simulink library "tenneco_lib"  (R2016b)
settings: Solver=ode45  StartTime=0.0  StopTime=10.0  RelTol=1e-3
undefined symbols (not defined in the file): Com_cntAMBInitTO_c, Com_cntAMBStopTO_c, Com_cntEC1InitTO_c, Com_cntEC1StopTO_c, Com_swAMBRx_c, Com_swEC1Rx_c, Com_swUseSPN108_c, Com_swUseSPN543_c, const, Env_pAmbPDflt_c, Env_pAmbPKOff_c, Env_pAmbPOvrd_c, Env_swAmbPOvrd_c, MSG_INIT_TIMEOUT, MSG_NOT_RECEIVED, MSG_RECEIVED_NOW, MSG_STOP_TIMEOUT
libraries: simulink x19, tenneco_lib x2
(part 2 of 5)

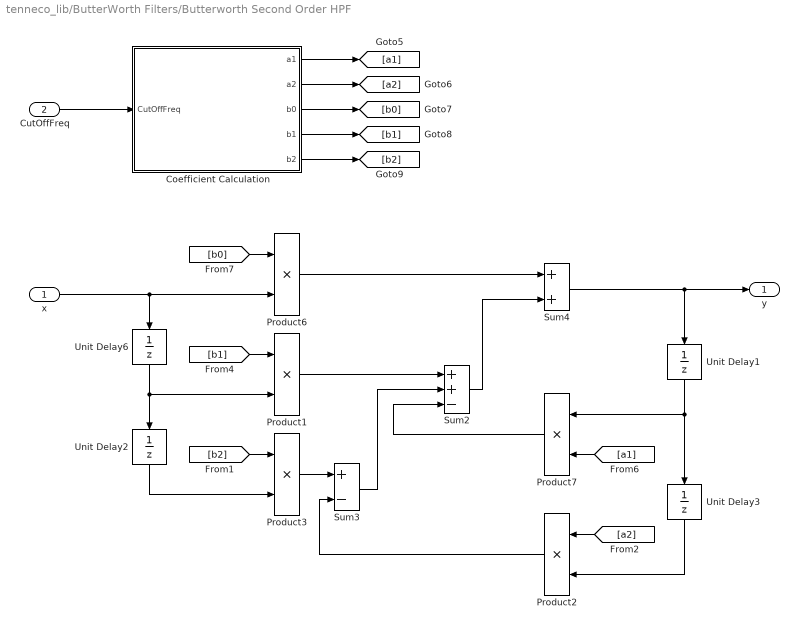
== system tenneco_lib/ButterWorth Filters/Butterworth Second Order HPF ==
  x : Inport  mask(Standard Inport){Port=1}
      mask prompts: Port "Simulink:blkprm_prompts:InOutportPortNum"
      mask help: Provide an input port for subsystems.
      mask TypeOptions Port: Port
  CutOffFreq : Inport  Port=2  mask(Standard Inport){Port=2}
      mask prompts: Port "Simulink:blkprm_prompts:InOutportPortNum"
      mask help: Provide an input port for subsystems.
      mask TypeOptions Port: Port
  Coefficient Calculation : Subsystem
  Product1 : Product  Inputs=**  InputSameDT=on  mask(Product){Inputs=**}
      mask prompts: Inputs "List of signs:"
      mask help:
      | Multiply or divide inputs.  Specify one of the following:
      |  a) * or / for each input port. For example, **/* performs the operation 'u1*u2/u3*u4'.
      |  b) scalar specifies the number of input ports to be multiplied.
      mask TypeOptions Inputs: Inputs
  Product2 : Product  Inputs=**  InputSameDT=on  mask(Product){Inputs=**}
      mask prompts: Inputs "List of signs:"
      mask help:
      | Multiply or divide inputs.  Specify one of the following:
      |  a) * or / for each input port. For example, **/* performs the operation 'u1*u2/u3*u4'.
      |  b) scalar specifies the number of input ports to be multiplied.
      mask TypeOptions Inputs: Inputs
  Product3 : Product  Inputs=**  InputSameDT=on  mask(Product){Inputs=**}
      mask prompts: Inputs "List of signs:"
      mask help:
      | Multiply or divide inputs.  Specify one of the following:
      |  a) * or / for each input port. For example, **/* performs the operation 'u1*u2/u3*u4'.
      |  b) scalar specifies the number of input ports to be multiplied.
      mask TypeOptions Inputs: Inputs
  Product6 : Product  Inputs=**  InputSameDT=on  mask(Product){Inputs=**}
      mask prompts: Inputs "List of signs:"
      mask help:
      | Multiply or divide inputs.  Specify one of the following:
      |  a) * or / for each input port. For example, **/* performs the operation 'u1*u2/u3*u4'.
      |  b) scalar specifies the number of input ports to be multiplied.
      mask TypeOptions Inputs: Inputs
  Product7 : Product  Inputs=**  InputSameDT=on  mask(Product){Inputs=**}
      mask prompts: Inputs "List of signs:"
      mask help:
      | Multiply or divide inputs.  Specify one of the following:
      |  a) * or / for each input port. For example, **/* performs the operation 'u1*u2/u3*u4'.
      |  b) scalar specifies the number of input ports to be multiplied.
      mask TypeOptions Inputs: Inputs
  Sum2 : Sum  Inputs=++-  InputSameDT=on  mask(Sum){Inputs=++-}
      mask prompts: Inputs "Simulink:blkprm_prompts:SumListofSigns"
      mask help:
      | Add or subtract inputs.  Specify one of the following:
      | a) character vector containing + or - for each input port, | for spacer between ports (e.g. ++|-|++)
      | b) scalar, >= 1, specifies the number of input ports to be summed.
      | When there is only one input port, add or subtract elements over all dimensions or one specified dimension
      mask TypeOptions Inputs: Inputs
  Sum3 : Sum  Inputs=+-  InputSameDT=on  mask(Sum){Inputs=+-}
      mask prompts: Inputs "Simulink:blkprm_prompts:SumListofSigns"
      mask help:
      | Add or subtract inputs.  Specify one of the following:
      | a) character vector containing + or - for each input port, | for spacer between ports (e.g. ++|-|++)
      | b) scalar, >= 1, specifies the number of input ports to be summed.
      | When there is only one input port, add or subtract elements over all dimensions or one specified dimension
      mask TypeOptions Inputs: Inputs
  Sum4 : Sum  InputSameDT=on  mask(Sum){Inputs=++}
      mask prompts: Inputs "Simulink:blkprm_prompts:SumListofSigns"
      mask help:
      | Add or subtract inputs.  Specify one of the following:
      | a) character vector containing + or - for each input port, | for spacer between ports (e.g. ++|-|++)
      | b) scalar, >= 1, specifies the number of input ports to be summed.
      | When there is only one input port, add or subtract elements over all dimensions or one specified dimension
      mask TypeOptions Inputs: Inputs
  Unit Delay1 : UnitDelay  InitialCondition=InitialCondition  SampleTime=-1  mask(Unit Delay){InitialCondition=0}
      mask prompts: InitialCondition "Simulink:blkprm_prompts:DelayBlkInitCond"
      mask help: Sample and hold with one sample period delay.
      mask TypeOptions InitialCondition: InitialCondition
  Unit Delay2 : UnitDelay  InitialCondition=InitialCondition  SampleTime=-1  mask(Unit Delay){InitialCondition=0}
      mask prompts: InitialCondition "Simulink:blkprm_prompts:DelayBlkInitCond"
      mask help: Sample and hold with one sample period delay.
      mask TypeOptions InitialCondition: InitialCondition
  Unit Delay3 : UnitDelay  InitialCondition=InitialCondition  SampleTime=-1  mask(Unit Delay){InitialCondition=0}
      mask prompts: InitialCondition "Simulink:blkprm_prompts:DelayBlkInitCond"
      mask help: Sample and hold with one sample period delay.
      mask TypeOptions InitialCondition: InitialCondition
  Unit Delay6 : UnitDelay  InitialCondition=InitialCondition  SampleTime=-1  mask(Unit Delay){InitialCondition=0}
      mask prompts: InitialCondition "Simulink:blkprm_prompts:DelayBlkInitCond"
      mask help: Sample and hold with one sample period delay.
      mask TypeOptions InitialCondition: InitialCondition
  y : Outport  mask(Standard Outport){Port=1}
      mask prompts: Port "Simulink:blkprm_prompts:InOutportPortNum"
      mask help: Provide an output port for subsystems.
      mask TypeOptions Port: Port
  wires:
  Unit Delay3/1 -> Product2/2
  Product2/1 -> Sum3/2
  [a2] -> Product2/1
  Sum3/1 -> Sum2/2
  Product3/1 -> Sum3/1
  Product7/1 -> Sum2/3
  Unit Delay2/1 -> Product3/2
  [b2] -> Product3/1
  Coefficient Calculation/5(b2) -> [b2]
  Coefficient Calculation/2(a2) -> [a2]
  CutOffFreq/1 -> Coefficient Calculation/1(CutOffFreq)
  x/1 -> Product6/2, Unit Delay6/1
  Coefficient Calculation/1(a1) -> [a1]
  Coefficient Calculation/4(b1) -> [b1]
  Coefficient Calculation/3(b0) -> [b0]
  Product6/1 -> Sum4/1
  Unit Delay6/1 -> Unit Delay2/1, Product1/2
  [b1] -> Product1/1
  [b0] -> Product6/1
  Product1/1 -> Sum2/1
  Sum2/1 -> Sum4/2
  [a1] -> Product7/2
  Unit Delay1/1 -> Product7/1, Unit Delay3/1
  Sum4/1 -> y/1, Unit Delay1/1

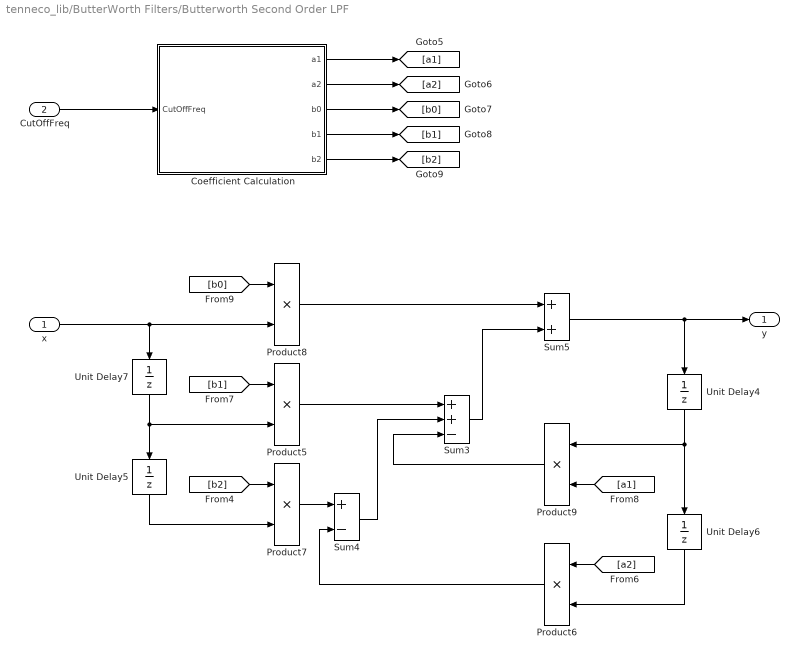
== system tenneco_lib/ButterWorth Filters/Butterworth Second Order LPF ==
  x : Inport  mask(Standard Inport){Port=1}
      mask prompts: Port "Simulink:blkprm_prompts:InOutportPortNum"
      mask help: Provide an input port for subsystems.
      mask TypeOptions Port: Port
  CutOffFreq : Inport  Port=2  mask(Standard Inport){Port=2}
      mask prompts: Port "Simulink:blkprm_prompts:InOutportPortNum"
      mask help: Provide an input port for subsystems.
      mask TypeOptions Port: Port
  Coefficient Calculation : Subsystem
  Product5 : Product  Inputs=**  InputSameDT=on  mask(Product){Inputs=**}
      mask prompts: Inputs "List of signs:"
      mask help:
      | Multiply or divide inputs.  Specify one of the following:
      |  a) * or / for each input port. For example, **/* performs the operation 'u1*u2/u3*u4'.
      |  b) scalar specifies the number of input ports to be multiplied.
      mask TypeOptions Inputs: Inputs
  Product6 : Product  Inputs=**  InputSameDT=on  mask(Product){Inputs=**}
      mask prompts: Inputs "List of signs:"
      mask help:
      | Multiply or divide inputs.  Specify one of the following:
      |  a) * or / for each input port. For example, **/* performs the operation 'u1*u2/u3*u4'.
      |  b) scalar specifies the number of input ports to be multiplied.
      mask TypeOptions Inputs: Inputs
  Product7 : Product  Inputs=**  InputSameDT=on  mask(Product){Inputs=**}
      mask prompts: Inputs "List of signs:"
      mask help:
      | Multiply or divide inputs.  Specify one of the following:
      |  a) * or / for each input port. For example, **/* performs the operation 'u1*u2/u3*u4'.
      |  b) scalar specifies the number of input ports to be multiplied.
      mask TypeOptions Inputs: Inputs
  Product8 : Product  Inputs=**  InputSameDT=on  mask(Product){Inputs=**}
      mask prompts: Inputs "List of signs:"
      mask help:
      | Multiply or divide inputs.  Specify one of the following:
      |  a) * or / for each input port. For example, **/* performs the operation 'u1*u2/u3*u4'.
      |  b) scalar specifies the number of input ports to be multiplied.
      mask TypeOptions Inputs: Inputs
  Product9 : Product  Inputs=**  InputSameDT=on  mask(Product){Inputs=**}
      mask prompts: Inputs "List of signs:"
      mask help:
      | Multiply or divide inputs.  Specify one of the following:
      |  a) * or / for each input port. For example, **/* performs the operation 'u1*u2/u3*u4'.
      |  b) scalar specifies the number of input ports to be multiplied.
      mask TypeOptions Inputs: Inputs
  Sum3 : Sum  Inputs=++-  InputSameDT=on  mask(Sum){Inputs=++-}
      mask prompts: Inputs "Simulink:blkprm_prompts:SumListofSigns"
      mask help:
      | Add or subtract inputs.  Specify one of the following:
      | a) character vector containing + or - for each input port, | for spacer between ports (e.g. ++|-|++)
      | b) scalar, >= 1, specifies the number of input ports to be summed.
      | When there is only one input port, add or subtract elements over all dimensions or one specified dimension
      mask TypeOptions Inputs: Inputs
  Sum4 : Sum  Inputs=+-  InputSameDT=on  mask(Sum){Inputs=+-}
      mask prompts: Inputs "Simulink:blkprm_prompts:SumListofSigns"
      mask help:
      | Add or subtract inputs.  Specify one of the following:
      | a) character vector containing + or - for each input port, | for spacer between ports (e.g. ++|-|++)
      | b) scalar, >= 1, specifies the number of input ports to be summed.
      | When there is only one input port, add or subtract elements over all dimensions or one specified dimension
      mask TypeOptions Inputs: Inputs
  Sum5 : Sum  InputSameDT=on  mask(Sum){Inputs=++}
      mask prompts: Inputs "Simulink:blkprm_prompts:SumListofSigns"
      mask help:
      | Add or subtract inputs.  Specify one of the following:
      | a) character vector containing + or - for each input port, | for spacer between ports (e.g. ++|-|++)
      | b) scalar, >= 1, specifies the number of input ports to be summed.
      | When there is only one input port, add or subtract elements over all dimensions or one specified dimension
      mask TypeOptions Inputs: Inputs
  Unit Delay4 : UnitDelay  InitialCondition=InitialCondition  SampleTime=-1  mask(Unit Delay){InitialCondition=0}
      mask prompts: InitialCondition "Simulink:blkprm_prompts:DelayBlkInitCond"
      mask help: Sample and hold with one sample period delay.
      mask TypeOptions InitialCondition: InitialCondition
  Unit Delay5 : UnitDelay  InitialCondition=InitialCondition  SampleTime=-1  mask(Unit Delay){InitialCondition=0}
      mask prompts: InitialCondition "Simulink:blkprm_prompts:DelayBlkInitCond"
      mask help: Sample and hold with one sample period delay.
      mask TypeOptions InitialCondition: InitialCondition
  Unit Delay6 : UnitDelay  InitialCondition=InitialCondition  SampleTime=-1  mask(Unit Delay){InitialCondition=0}
      mask prompts: InitialCondition "Simulink:blkprm_prompts:DelayBlkInitCond"
      mask help: Sample and hold with one sample period delay.
      mask TypeOptions InitialCondition: InitialCondition
  Unit Delay7 : UnitDelay  InitialCondition=InitialCondition  SampleTime=-1  mask(Unit Delay){InitialCondition=0}
      mask prompts: InitialCondition "Simulink:blkprm_prompts:DelayBlkInitCond"
      mask help: Sample and hold with one sample period delay.
      mask TypeOptions InitialCondition: InitialCondition
  y : Outport  mask(Standard Outport){Port=1}
      mask prompts: Port "Simulink:blkprm_prompts:InOutportPortNum"
      mask help: Provide an output port for subsystems.
      mask TypeOptions Port: Port
  wires:
  CutOffFreq/1 -> Coefficient Calculation/1(CutOffFreq)
  Unit Delay6/1 -> Product6/2
  Product6/1 -> Sum4/2
  [a2] -> Product6/1
  Sum4/1 -> Sum3/2
  Product7/1 -> Sum4/1
  Product9/1 -> Sum3/3
  Unit Delay5/1 -> Product7/2
  [b2] -> Product7/1
  Coefficient Calculation/5(b2) -> [b2]
  Coefficient Calculation/2(a2) -> [a2]
  x/1 -> Product8/2, Unit Delay7/1
  Coefficient Calculation/1(a1) -> [a1]
  Coefficient Calculation/4(b1) -> [b1]
  Coefficient Calculation/3(b0) -> [b0]
  Product8/1 -> Sum5/1
  Unit Delay7/1 -> Unit Delay5/1, Product5/2
  [b1] -> Product5/1
  [b0] -> Product8/1
  Product5/1 -> Sum3/1
  Sum3/1 -> Sum5/2
  [a1] -> Product9/2
  Unit Delay4/1 -> Product9/1, Unit Delay6/1
  Sum5/1 -> y/1, Unit Delay4/1

== system tenneco_lib/ButterWorth Filters/Generic Low-Pass Filter ==
  In : Inport  mask(Standard Inport){Port=1}
      mask prompts: Port "Simulink:blkprm_prompts:InOutportPortNum"
      mask help: Provide an input port for subsystems.
      mask TypeOptions Port: Port
  Constant1 : Constant  Value=Value  mask(Constant){Value=Fil}
      mask prompts: Value "Simulink:blkprm_prompts:ConstConstValue"
      mask help: Output the constant specified by the 'Constant value' parameter. If 'Constant value' is a vector, treat the constant value as a 1-D array.
      mask init: same as tenneco_lib/Sources/Constant
      mask TypeOptions Value: Value
      mask Display: disp(str)
  Product1 : Product  Inputs=**  InputSameDT=on  mask(Product){Inputs=**}
      mask prompts: Inputs "List of signs:"
      mask help:
      | Multiply or divide inputs.  Specify one of the following:
      |  a) * or / for each input port. For example, **/* performs the operation 'u1*u2/u3*u4'.
      |  b) scalar specifies the number of input ports to be multiplied.
      mask TypeOptions Inputs: Inputs
  Stabilize Counter : Subsystem
  Sum1 : Sum  Inputs=+-  InputSameDT=on  mask(Sum){Inputs=+-}
      mask prompts: Inputs "Simulink:blkprm_prompts:SumListofSigns"
      mask help:
      | Add or subtract inputs.  Specify one of the following:
      | a) character vector containing + or - for each input port, | for spacer between ports (e.g. ++|-|++)
      | b) scalar, >= 1, specifies the number of input ports to be summed.
      | When there is only one input port, add or subtract elements over all dimensions or one specified dimension
      mask TypeOptions Inputs: Inputs
  Sum2 : Sum  InputSameDT=on  mask(Sum){Inputs=++}
      mask prompts: Inputs "Simulink:blkprm_prompts:SumListofSigns"
      mask help:
      | Add or subtract inputs.  Specify one of the following:
      | a) character vector containing + or - for each input port, | for spacer between ports (e.g. ++|-|++)
      | b) scalar, >= 1, specifies the number of input ports to be summed.
      | When there is only one input port, add or subtract elements over all dimensions or one specified dimension
      mask TypeOptions Inputs: Inputs
  Switch1 : Switch  Threshold=0.5  mask(Switch){}
      mask help: Pass through input 1 when input 2 satisfies the selected criterion; otherwise, pass through input 3. The inputs are numbered top to bottom (or left to right). The first and third input ports are data ports, and the second input port is the control port. The criteria for control port 2 are u2 >= Threshold (0.5).
  Unit Delay1 : UnitDelay  InitialCondition=InitialCondition  SampleTime=-1  mask(Unit Delay){InitialCondition=0}
      mask prompts: InitialCondition "Simulink:blkprm_prompts:DelayBlkInitCond"
      mask help: Sample and hold with one sample period delay.
      mask TypeOptions InitialCondition: InitialCondition
  Out : Outport  mask(Standard Outport){Port=1}
      mask prompts: Port "Simulink:blkprm_prompts:InOutportPortNum"
      mask help: Provide an output port for subsystems.
      mask TypeOptions Port: Port
  wires:
  In/1 -> Switch1/1, Sum1/1
  Unit Delay1/1 -> Sum1/2, Sum2/2
  Sum1/1 -> Product1/2
  Constant1/1 -> Product1/1
  Product1/1 -> Sum2/1
  Sum2/1 -> Switch1/3
  Switch1/1 -> Out/1, Unit Delay1/1
  Stabilize Counter/1(Stable) -> Switch1/2

== system tenneco_lib/ButterWorth Filters/Resettable Variable Low-Pass Filter ==
  note: Note : Simulink constant block used because Tenneco constant block is not generic and datatype friendly
  In : Inport  mask(Standard Inport){Port=1}
      mask prompts: Port "Simulink:blkprm_prompts:InOutportPortNum"
      mask help: Provide an input port for subsystems.
      mask TypeOptions Port: Port
  Tau : Inport  Port=2  mask(Standard Inport){Port=2}
      mask prompts: Port "Simulink:blkprm_prompts:InOutportPortNum"
      mask help: Provide an input port for subsystems.
      mask TypeOptions Port: Port
  Reset : Inport  Port=3  mask(Standard Inport){Port=3}
      mask prompts: Port "Simulink:blkprm_prompts:InOutportPortNum"
      mask help: Provide an input port for subsystems.
      mask TypeOptions Port: Port
  Constant9 : Constant  Value=Ts  OutDataTypeStr=Inherit: Inherit via back propagation
  Logical Operator1 : Logic  Operator=NOT  Inputs=Inputs  AllPortsSameDT=off  OutDataTypeStr=boolean  mask(Logical Operator){Operator=NOT, Inputs=2}
      mask prompts: Operator "Simulink:blkprm_prompts:LogicOperator"; Inputs "Simulink:blkprm_prompts:LogicNumInputPorts"
      mask help: Logical operators. For a single input, operators are applied across the input vector. For multiple inputs, operators are applied across the inputs.
      mask TypeOptions Operator: Operator
      mask TypeOptions Inputs: Inputs
  Logical Operator2 : Logic  Inputs=Inputs  AllPortsSameDT=off  OutDataTypeStr=boolean  mask(Logical Operator){Operator=AND, Inputs=2}
      mask prompts: Operator "Simulink:blkprm_prompts:LogicOperator"; Inputs "Simulink:blkprm_prompts:LogicNumInputPorts"
      mask help: Logical operators. For a single input, operators are applied across the input vector. For multiple inputs, operators are applied across the inputs.
      mask TypeOptions Operator: Operator
      mask TypeOptions Inputs: Inputs
  Product1 : Product  Inputs=*/  InputSameDT=on  mask(Product){Inputs=*/}
      mask prompts: Inputs "List of signs:"
      mask help:
      | Multiply or divide inputs.  Specify one of the following:
      |  a) * or / for each input port. For example, **/* performs the operation 'u1*u2/u3*u4'.
      |  b) scalar specifies the number of input ports to be multiplied.
      mask TypeOptions Inputs: Inputs
  Product2 : Product  Inputs=**  InputSameDT=on  mask(Product){Inputs=**}
      mask prompts: Inputs "List of signs:"
      mask help:
      | Multiply or divide inputs.  Specify one of the following:
      |  a) * or / for each input port. For example, **/* performs the operation 'u1*u2/u3*u4'.
      |  b) scalar specifies the number of input ports to be multiplied.
      mask TypeOptions Inputs: Inputs
  Saturation1 : Saturate  UpperLimit=UpperLimit  LowerLimit=LowerLimit  mask(Saturation){UpperLimit=Inf, LowerLimit=Ts}
      mask prompts: UpperLimit "Simulink:blkprm_prompts:SaturateUpLim"; LowerLimit "Simulink:blkprm_prompts:SaturateLowLim"
      mask help: Limit input signal to the upper and lower saturation values.
      mask TypeOptions UpperLimit: UpperLimit
      mask TypeOptions LowerLimit: LowerLimit
  Stabilize Counter : Subsystem
  Sum : Sum  Inputs=-+  InputSameDT=on  mask(Sum){Inputs=-+}
      mask prompts: Inputs "Simulink:blkprm_prompts:SumListofSigns"
      mask help:
      | Add or subtract inputs.  Specify one of the following:
      | a) character vector containing + or - for each input port, | for spacer between ports (e.g. ++|-|++)
      | b) scalar, >= 1, specifies the number of input ports to be summed.
      | When there is only one input port, add or subtract elements over all dimensions or one specified dimension
      mask TypeOptions Inputs: Inputs
  Sum2 : Sum  InputSameDT=on  mask(Sum){Inputs=++}
      mask prompts: Inputs "Simulink:blkprm_prompts:SumListofSigns"
      mask help:
      | Add or subtract inputs.  Specify one of the following:
      | a) character vector containing + or - for each input port, | for spacer between ports (e.g. ++|-|++)
      | b) scalar, >= 1, specifies the number of input ports to be summed.
      | When there is only one input port, add or subtract elements over all dimensions or one specified dimension
      mask TypeOptions Inputs: Inputs
  Switch : Switch  Threshold=0.5  mask(Switch){}
      mask help: Pass through input 1 when input 2 satisfies the selected criterion; otherwise, pass through input 3. The inputs are numbered top to bottom (or left to right). The first and third input ports are data ports, and the second input port is the control port. The criteria for control port 2 are u2 >= Threshold (0.5).
  Unit Delay1 : UnitDelay  InitialCondition=InitialCondition  SampleTime=-1  mask(Unit Delay){InitialCondition=0}
      mask prompts: InitialCondition "Simulink:blkprm_prompts:DelayBlkInitCond"
      mask help: Sample and hold with one sample period delay.
      mask TypeOptions InitialCondition: InitialCondition
  Out : Outport  mask(Standard Outport){Port=1}
      mask prompts: Port "Simulink:blkprm_prompts:InOutportPortNum"
      mask help: Provide an output port for subsystems.
      mask TypeOptions Port: Port
  wires:
  Product1/1 -> Product2/2
  Sum2/1 -> Switch/1
  Sum/1 -> Product2/1
  Product2/1 -> Sum2/2
  Switch/1 -> Out/1, Unit Delay1/1
  Unit Delay1/1 -> Sum/1, Sum2/1
  In/1 -> Switch/3, Sum/2
  Constant9/1 -> Product1/1
  Tau/1 -> Saturation1/1
  Saturation1/1 -> Product1/2
  Reset/1 -> Logical Operator1/1
  Stabilize Counter/1(Stable) -> Logical Operator2/1
  Logical Operator1/1 -> Logical Operator2/2
  Logical Operator2/1 -> Switch/2

== system tenneco_lib/ButterWorth Filters/Variable Low-Pass Filter ==
  note: Note : Simulink constant block used because Tenneco constant block is not generic and datatype friendly
  In : Inport  mask(Standard Inport){Port=1}
      mask prompts: Port "Simulink:blkprm_prompts:InOutportPortNum"
      mask help: Provide an input port for subsystems.
      mask TypeOptions Port: Port
  Tau : Inport  Port=2  mask(Standard Inport){Port=2}
      mask prompts: Port "Simulink:blkprm_prompts:InOutportPortNum"
      mask help: Provide an input port for subsystems.
      mask TypeOptions Port: Port
  Constant9 : Constant  Value=Ts  OutDataTypeStr=Inherit: Inherit via back propagation
  Product1 : Product  Inputs=*/  InputSameDT=on  mask(Product){Inputs=*/}
      mask prompts: Inputs "List of signs:"
      mask help:
      | Multiply or divide inputs.  Specify one of the following:
      |  a) * or / for each input port. For example, **/* performs the operation 'u1*u2/u3*u4'.
      |  b) scalar specifies the number of input ports to be multiplied.
      mask TypeOptions Inputs: Inputs
  Product2 : Product  Inputs=**  InputSameDT=on  mask(Product){Inputs=**}
      mask prompts: Inputs "List of signs:"
      mask help:
      | Multiply or divide inputs.  Specify one of the following:
      |  a) * or / for each input port. For example, **/* performs the operation 'u1*u2/u3*u4'.
      |  b) scalar specifies the number of input ports to be multiplied.
      mask TypeOptions Inputs: Inputs
  Saturation1 : Saturate  UpperLimit=UpperLimit  LowerLimit=LowerLimit  mask(Saturation){UpperLimit=inf, LowerLimit=Ts}
      mask prompts: UpperLimit "Simulink:blkprm_prompts:SaturateUpLim"; LowerLimit "Simulink:blkprm_prompts:SaturateLowLim"
      mask help: Limit input signal to the upper and lower saturation values.
      mask TypeOptions UpperLimit: UpperLimit
      mask TypeOptions LowerLimit: LowerLimit
  Stabilize Counter : Subsystem
  Sum : Sum  Inputs=-+  InputSameDT=on  mask(Sum){Inputs=-+}
      mask prompts: Inputs "Simulink:blkprm_prompts:SumListofSigns"
      mask help:
      | Add or subtract inputs.  Specify one of the following:
      | a) character vector containing + or - for each input port, | for spacer between ports (e.g. ++|-|++)
      | b) scalar, >= 1, specifies the number of input ports to be summed.
      | When there is only one input port, add or subtract elements over all dimensions or one specified dimension
      mask TypeOptions Inputs: Inputs
  Sum2 : Sum  InputSameDT=on  mask(Sum){Inputs=++}
      mask prompts: Inputs "Simulink:blkprm_prompts:SumListofSigns"
      mask help:
      | Add or subtract inputs.  Specify one of the following:
      | a) character vector containing + or - for each input port, | for spacer between ports (e.g. ++|-|++)
      | b) scalar, >= 1, specifies the number of input ports to be summed.
      | When there is only one input port, add or subtract elements over all dimensions or one specified dimension
      mask TypeOptions Inputs: Inputs
  Switch : Switch  Threshold=0.5  mask(Switch){}
      mask help: Pass through input 1 when input 2 satisfies the selected criterion; otherwise, pass through input 3. The inputs are numbered top to bottom (or left to right). The first and third input ports are data ports, and the second input port is the control port. The criteria for control port 2 are u2 >= Threshold (0.5).
  Unit Delay1 : UnitDelay  InitialCondition=InitialCondition  SampleTime=-1  mask(Unit Delay){InitialCondition=0}
      mask prompts: InitialCondition "Simulink:blkprm_prompts:DelayBlkInitCond"
      mask help: Sample and hold with one sample period delay.
      mask TypeOptions InitialCondition: InitialCondition
  Out : Outport  mask(Standard Outport){Port=1}
      mask prompts: Port "Simulink:blkprm_prompts:InOutportPortNum"
      mask help: Provide an output port for subsystems.
      mask TypeOptions Port: Port
  wires:
  Saturation1/1 -> Product1/2
  Tau/1 -> Saturation1/1
  Constant9/1 -> Product1/1
  In/1 -> Switch/3, Sum/2
  Unit Delay1/1 -> Sum/1, Sum2/1
  Switch/1 -> Unit Delay1/1, Out/1
  Stabilize Counter/1(Stable) -> Switch/2
  Product2/1 -> Sum2/2
  Sum/1 -> Product2/1
  Sum2/1 -> Switch/1
  Product1/1 -> Product2/2

== system tenneco_lib/Custom/CAN ==
  Generic CAN Input : Subsystem  mask(Generic Input){RATE=1.0, CAN_CNT_INIT=Com_cntAMBInitTO_c, CAN_CNT_STOP=Com_cntAMBStopTO_c, CAN_OOR_VALUE=64255, CAN_RECV_SW=Com_swAMBRx_c, CAN_USE_SW=Com_swUseSPN108_c, MAN_OVRD_VALUE=Env_pAmbPOvrd_c, MAN_OVRD_SW=Env_swAmbPOvrd_c, KEY_OFF_VALUE=Env_pAmbPKOff_c, DEFAULT_VALUE=Env_pAmbPDflt_c, SLOPE=(1/2), OFFSET=0}
      mask prompts: RATE "Task Rate"; CAN_CNT_INIT "CAN init count"; CAN_CNT_STOP "CAN stop count"; CAN_OOR_VALUE "CAN OOR value"; CAN_RECV_SW "CAN receive switch"; CAN_USE_SW "CAN use switch"; MAN_OVRD_VALUE "Manual override value"; MAN_OVRD_SW "Manual override switch"; KEY_OFF_VALUE "Key off default value"; DEFAULT_VALUE "Default value ( if CAN invalid)"; SLOPE "Data slope (multiply by)"; OFFSET "Data offset (add to)"
      mask help: Takes the analog and CAN raw data and converts it into a usable value.
      mask Display:
      | image(imread('Tenneco_Copyright_Logo_Mini.bmp'),'center');
      | color('red');
      | disp('\n\n\n\n\n\n\nTenneco Confidential Red\n Restricted. Do not Distribute.');
  Generic Valueless CAN Input : Subsystem  mask(Generic Input){RATE=0.5, CAN_CNT_INIT=Com_cntEC1InitTO_c, CAN_CNT_STOP=Com_cntEC1StopTO_c, CAN_OOR_VALUE=256, CAN_RECV_SW=Com_swEC1Rx_c, CAN_USE_SW=Com_swUseSPN543_c}
      mask prompts: RATE "Task Rate"; CAN_CNT_INIT "CAN init count"; CAN_CNT_STOP "CAN stop count"; CAN_OOR_VALUE "CAN OOR value"; CAN_RECV_SW "CAN receive switch"; CAN_USE_SW "CAN use switch"
      mask help: Takes the analog and CAN raw data and converts it into a usable value.
      mask Display:
      | image(imread('Tenneco_Copyright_Logo_Mini.bmp'),'center');
      | color('red');
      | disp('\n\n\n\n\n\n\nTenneco Confidential Red\n Restricted. Do not Distribute.');
  Timeout Check : Subsystem  mask(CAN Timeout){}
      mask help: Determines timeout for CAN
      mask Display:
      | image(imread('Tenneco_Copyright_Logo_Mini.bmp'),'center');
      | color('red');
      | disp('\n\n\n\n\n\n\nTenneco Confidential Red\n Restricted. Do not Distribute.');

== system tenneco_lib/Custom/Logical ==
  Latch : Subsystem  TreatAsAtomicUnit=on  mask(Latch){INIT=0}
      mask prompts: INIT "Initial Value:"
      mask help:
      | Provide conditions to 'Set' input to latch the output to 1.
      |
      | The output will remain 1 until the conditions at the 'Reset input are true, at which point the output will go to zero.
      |
      | An initial value may be entered but must be either 0 or 1.
      mask Display:
      | image(imread('Tenneco_Copyright_Logo_Mini.bmp'),'center');
      | color('red');
      | disp('\n\n\n\n\n\n\nTenneco Confidential Red\n Restricted. Do not Distribute.');

== system tenneco_lib/Custom/Math ==
  Divide by zero protection : Subsystem  TreatAsAtomicUnit=on  mask{default=1}
      mask prompts: default "Output when denominator is zero"
      mask Display:
      | port_label('input',1,' x');
      | port_label('input',2,' /');
      | port_label('output',1,'Out');
      | image(imread('Tenneco_Copyright_Logo_Mini.bmp'),'center');
      | color('red');
      | disp('\n\n\n\n\n\n\nTenneco Confidential Red\n Restricted. Do not Distribute.');
  Time_Based_Rate_Limiter : Subsystem  TreatAsAtomicUnit=on  mask(Rate Limiter){Fs=200}
      mask prompts: Fs "sample frequency(Hz)"
      mask help: Assign rise time and fall time to adjust the change of input
      mask Display:
      | image(imread('Tenneco_Copyright_Logo_Mini.bmp'),'center');
      | color('red');
      | disp('\n\n\n\n\n\n\nTenneco Confidential Red\n Restricted. Do not Distribute.');

== system tenneco_lib/Custom/Timers ==
  Delay_Time : Subsystem  TreatAsAtomicUnit=on  mask(DELAY_TIME){}
      mask help:
      | If "condition" is TRUE
      | {
      |     then "delay_act" will be FALSE for the time "delay_t" and then become TRUE after "delay_t" time is expired.
      | }
      |
      | else
      | {
      |     "delay_act" is always FALSE.
      | }
      |
      | step_time = execution  rate
      mask Display:
      | image(imread('Tenneco_Copyright_Logo_Mini.bmp'),'center');
      | color('red');
      | disp('\n\n\n\n\n\n\nTenneco Confidential Red\n Restricted. Do not Distribute.');
  Hold_Time : Subsystem  TreatAsAtomicUnit=on  mask(HOLD_TIME){}
      mask help:
      | If "condition" is TRUE
      | {
      |     then "hold_active" will be TRUE
      | }
      |
      | else
      | {
      |     If timer counter < time "hold_t"
      |     {
      |         then "hold_active" will be TRUE for the time "hold_t" and then become FALSE after "hold_t" time is expired.
      |     }
      |
      |     else
      |     {
      |         "hold_active" is always FALSE.
      |     }
      | }
      mask Display:
      | image(imread('Tenneco_Copyright_Logo_Mini.bmp'),'center');
      | color('red');
      | disp('\n\n\n\n\n\n\nTenneco Confidential Red\n Restricted. Do not Distribute.');
  Timer/Counter : Subsystem  TreatAsAtomicUnit=on  mask(Timer/Counter){INIT=0, INC_STEP=0.1, DEC_STEP=0}
      mask prompts: INIT "Initial Value:"; INC_STEP "Increment Step:"; DEC_STEP "Decrement Step:"
      mask help:
      | This block may be used as a timer or a counter. Conditions for each action should be provided to the respective inputs.
      |
      | The user can specify an initial value. The initial value is also the value that the output will return to upon reset.
      |
      | Separate step values can be specified by the user for incrementing and decrementing. The step value is based on the subsystem loop rate.
      mask Display:
      | image(imread('Tenneco_Copyright_Logo_Mini.bmp'),'center');
      | color('red');
      | disp('\n\n\n\n\n\n\nTenneco Confidential Red\n Restricted. Do not Distribute.');

== system tenneco_lib/Model Documentation/Appendix Title ==
  Description1 : Subsystem  mask(RptGenDescription){rptgenOrder=20}
      mask prompts: rptgenOrder "Report Gen Order Priority"
      mask help:
      | This block can contain text, tables, lists, images, and equations from a Word document to describe its parent subsystem.
      |
      | The contents of this block shall be placed in paragraph(s) just after the subsystem's section heading in the report, before the system snapshot.
      |
      | The Report Gen Order Priority allows the user to set the sorted order of the block's contents appearing in the report.
      settings: OpenFcn=open_system([gcb,'/DocBlock'])
      mask Display: disp(['Description - ',get_param(gcb,'rptgenOrder')])

== system tenneco_lib/Model Documentation/Description ==
  DocBlock : simulink/Model-Wide Utilities/DocBlock  DocumentType=RTF

== system tenneco_lib/Model Documentation/Detail ==
  DocBlock : simulink/Model-Wide Utilities/DocBlock  DocumentType=RTF

== system tenneco_lib/Model Documentation/Introduction ==
  DocBlock : simulink/Model-Wide Utilities/DocBlock  DocumentType=RTF

== system tenneco_lib/Ports & Subsystems/If Action Subsystem ==
  In1 : Inport  mask(Standard Inport){Port=1}
      mask prompts: Port "Simulink:blkprm_prompts:InOutportPortNum"
      mask help: Provide an input port for subsystems.
      settings: CopyFcn=set_param(gcbh,'LinkStatus','none');
      mask TypeOptions Port: Port
  Action Port : ActionPort  ActionType=then
  Out1 : Outport  mask(Standard Outport){Port=1}
      mask prompts: Port "Simulink:blkprm_prompts:InOutportPortNum"
      mask help: Provide an output port for subsystems.
      settings: CopyFcn=set_param(gcbh,'LinkStatus','none');
      mask TypeOptions Port: Port
  wires:
  In1/1 -> Out1/1

== system tenneco_lib/Ports & Subsystems/SoftwareComponent SWC ==
  Root_Level_Inport : Inport  OutMin=OutMin  OutMax=OutMax  Unit=m/s  PortDimensions=1  SampleTime=SampleTime  mask(Root Level Inport){Port=1, OutDataTypeStr=Inherit: auto, PortDimensions=1, Resolution=0.001, OutMin=-10, OutMax=10, Unit=m/s, SampleTime=-1, varSource=SoftwarePart_dd}
      mask prompts: Port "Simulink:blkprm_prompts:InOutportPortNum"; OutDataTypeStr "Simulink:blkprm_prompts:UNIFIEDDATATYPE"; PortDimensions "Simulink:blkprm_prompts:InportPortDims"; OutMin "Simulink:blkprm_prompts:DesignMin"; OutMax "Simulink:blkprm_prompts:DesignMax"; Unit "Simulink:blkprm_prompts:OutputUnit_EditField"; SampleTime "Simulink:blkprm_prompts:AllBlksSampleTime"; varSource "Signal Source"
      mask help:
      | Provide an input port for a software component.
      |
      | The data type, dimensions, and engineering units should be defined to detect mismatched properties to connected signals, and for design document generatioin.
      |
      | Minimum, maximum, and source should be filled in for report generation.
      settings: AttributesFormatString=%<Unit>  CopyFcn=set_param(gcbh,'LinkStatus','none');
      mask TypeOptions Port: Port
      mask TypeOptions OutDataTypeStr: OutDataTypeStr
      mask TypeOptions PortDimensions: PortDimensions
      mask TypeOptions OutMin: OutMin
      mask TypeOptions OutMax: OutMax
      mask TypeOptions Unit: Unit
      mask TypeOptions SampleTime: SampleTime
  Root Level Outport : Outport  OutMin=OutMin  OutMax=OutMax  SampleTime=SampleTime  mask(Root Level Outport){Port=1, OutDataTypeStr=Inherit: auto, PortDimensions=-1, SampleTime=-1, OutMin=[], OutMax=[], Unit=inherit}
      mask prompts: Port "Simulink:blkprm_prompts:InOutportPortNum"; OutDataTypeStr "Simulink:blkprm_prompts:UNIFIEDDATATYPE"; PortDimensions "Simulink:blkprm_prompts:InportPortDims"; SampleTime "Simulink:blkprm_prompts:AllBlksSampleTime"; OutMin "Simulink:blkprm_prompts:DesignMin"; OutMax "Simulink:blkprm_prompts:DesignMax"; Unit "Simulink:blkprm_prompts:OutputUnit_EditField"
      mask help: Provide a root level output port for a model.
      settings: CopyFcn=set_param(gcbh,'LinkStatus','none');
      mask TypeOptions Port: Port
      mask TypeOptions OutDataTypeStr: OutDataTypeStr
      mask TypeOptions PortDimensions: PortDimensions
      mask TypeOptions SampleTime: SampleTime
      mask TypeOptions OutMin: OutMin
      mask TypeOptions OutMax: OutMax
      mask TypeOptions Unit: Unit
  wires:
  Root_Level_Inport/1 -> Root Level Outport/1

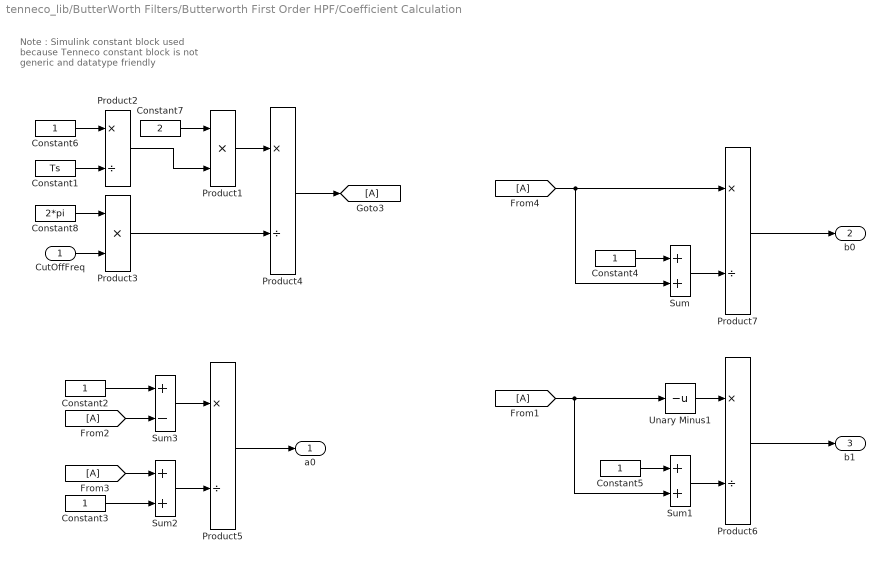
== system tenneco_lib/ButterWorth Filters/Butterworth First Order HPF/Coefficient Calculation ==
  note: Note : Simulink constant block used because Tenneco constant block is not generic and datatype friendly
  CutOffFreq : Inport  mask(Standard Inport){Port=1}
      mask prompts: Port "Simulink:blkprm_prompts:InOutportPortNum"
      mask help: Provide an input port for subsystems.
      mask TypeOptions Port: Port
  Constant1 : Constant  Value=Ts  OutDataTypeStr=Inherit: Inherit via back propagation
  Constant{2..6} (5 alike) : Constant  OutDataTypeStr=Inherit: Inherit via back propagation
  Constant7 : Constant  Value=2  OutDataTypeStr=Inherit: Inherit via back propagation
  Constant8 : Constant  Value=2*pi  OutDataTypeStr=Inherit: Inherit via back propagation
  Product1 : Product  Inputs=**  InputSameDT=on  mask(Product){Inputs=**}
      mask prompts: Inputs "List of signs:"
      mask help:
      | Multiply or divide inputs.  Specify one of the following:
      |  a) * or / for each input port. For example, **/* performs the operation 'u1*u2/u3*u4'.
      |  b) scalar specifies the number of input ports to be multiplied.
      mask TypeOptions Inputs: Inputs
  Product2 : Product  Inputs=*/  InputSameDT=on  mask(Product){Inputs=*/}
      mask prompts: Inputs "List of signs:"
      mask help:
      | Multiply or divide inputs.  Specify one of the following:
      |  a) * or / for each input port. For example, **/* performs the operation 'u1*u2/u3*u4'.
      |  b) scalar specifies the number of input ports to be multiplied.
      mask TypeOptions Inputs: Inputs
  Product3 : Product  Inputs=**  InputSameDT=on  mask(Product){Inputs=**}
      mask prompts: Inputs "List of signs:"
      mask help:
      | Multiply or divide inputs.  Specify one of the following:
      |  a) * or / for each input port. For example, **/* performs the operation 'u1*u2/u3*u4'.
      |  b) scalar specifies the number of input ports to be multiplied.
      mask TypeOptions Inputs: Inputs
  Product4 : Product  Inputs=*/  InputSameDT=on  mask(Product){Inputs=*/}
      mask prompts: Inputs "List of signs:"
      mask help:
      | Multiply or divide inputs.  Specify one of the following:
      |  a) * or / for each input port. For example, **/* performs the operation 'u1*u2/u3*u4'.
      |  b) scalar specifies the number of input ports to be multiplied.
      mask TypeOptions Inputs: Inputs
  Product5 : Product  Inputs=*/  InputSameDT=on  mask(Product){Inputs=*/}
      mask prompts: Inputs "List of signs:"
      mask help:
      | Multiply or divide inputs.  Specify one of the following:
      |  a) * or / for each input port. For example, **/* performs the operation 'u1*u2/u3*u4'.
      |  b) scalar specifies the number of input ports to be multiplied.
      mask TypeOptions Inputs: Inputs
  Product6 : Product  Inputs=*/  InputSameDT=on  mask(Product){Inputs=*/}
      mask prompts: Inputs "List of signs:"
      mask help:
      | Multiply or divide inputs.  Specify one of the following:
      |  a) * or / for each input port. For example, **/* performs the operation 'u1*u2/u3*u4'.
      |  b) scalar specifies the number of input ports to be multiplied.
      mask TypeOptions Inputs: Inputs
  Product7 : Product  Inputs=*/  InputSameDT=on  mask(Product){Inputs=*/}
      mask prompts: Inputs "List of signs:"
      mask help:
      | Multiply or divide inputs.  Specify one of the following:
      |  a) * or / for each input port. For example, **/* performs the operation 'u1*u2/u3*u4'.
      |  b) scalar specifies the number of input ports to be multiplied.
      mask TypeOptions Inputs: Inputs
  Sum : Sum  InputSameDT=on  mask(Sum){Inputs=++}
      mask prompts: Inputs "Simulink:blkprm_prompts:SumListofSigns"
      mask help:
      | Add or subtract inputs.  Specify one of the following:
      | a) character vector containing + or - for each input port, | for spacer between ports (e.g. ++|-|++)
      | b) scalar, >= 1, specifies the number of input ports to be summed.
      | When there is only one input port, add or subtract elements over all dimensions or one specified dimension
      mask TypeOptions Inputs: Inputs
  Sum1 : Sum  InputSameDT=on  mask(Sum){Inputs=++}
      mask prompts: Inputs "Simulink:blkprm_prompts:SumListofSigns"
      mask help:
      | Add or subtract inputs.  Specify one of the following:
      | a) character vector containing + or - for each input port, | for spacer between ports (e.g. ++|-|++)
      | b) scalar, >= 1, specifies the number of input ports to be summed.
      | When there is only one input port, add or subtract elements over all dimensions or one specified dimension
      mask TypeOptions Inputs: Inputs
  Sum2 : Sum  InputSameDT=on  mask(Sum){Inputs=++}
      mask prompts: Inputs "Simulink:blkprm_prompts:SumListofSigns"
      mask help:
      | Add or subtract inputs.  Specify one of the following:
      | a) character vector containing + or - for each input port, | for spacer between ports (e.g. ++|-|++)
      | b) scalar, >= 1, specifies the number of input ports to be summed.
      | When there is only one input port, add or subtract elements over all dimensions or one specified dimension
      mask TypeOptions Inputs: Inputs
  Sum3 : Sum  Inputs=+-  InputSameDT=on  mask(Sum){Inputs=+-}
      mask prompts: Inputs "Simulink:blkprm_prompts:SumListofSigns"
      mask help:
      | Add or subtract inputs.  Specify one of the following:
      | a) character vector containing + or - for each input port, | for spacer between ports (e.g. ++|-|++)
      | b) scalar, >= 1, specifies the number of input ports to be summed.
      | When there is only one input port, add or subtract elements over all dimensions or one specified dimension
      mask TypeOptions Inputs: Inputs
  Unary Minus1 : UnaryMinus
  a0 : Outport  mask(Standard Outport){Port=1}
      mask prompts: Port "Simulink:blkprm_prompts:InOutportPortNum"
      mask help: Provide an output port for subsystems.
      mask TypeOptions Port: Port
  b0 : Outport  Port=2  mask(Standard Outport){Port=2}
      mask prompts: Port "Simulink:blkprm_prompts:InOutportPortNum"
      mask help: Provide an output port for subsystems.
      mask TypeOptions Port: Port
  b1 : Outport  Port=3  mask(Standard Outport){Port=3}
      mask prompts: Port "Simulink:blkprm_prompts:InOutportPortNum"
      mask help: Provide an output port for subsystems.
      mask TypeOptions Port: Port
  wires:
  Constant7/1 -> Product1/1
  Product2/1 -> Product1/2
  Product1/1 -> Product4/1
  Product4/1 -> [A]
  Product3/1 -> Product4/2
  Constant8/1 -> Product3/1
  Constant6/1 -> Product2/1
  CutOffFreq/1 -> Product3/2
  Constant1/1 -> Product2/2
  Product6/1 -> b1/1
  Constant5/1 -> Sum1/1
  Sum1/1 -> Product6/2
  Unary Minus1/1 -> Product6/1
  [A] -> Sum1/2, Unary Minus1/1
  Product7/1 -> b0/1
  [A] -> Product7/1, Sum/2
  Constant4/1 -> Sum/1
  Sum/1 -> Product7/2
  Product5/1 -> a0/1
  Constant3/1 -> Sum2/2
  [A] -> Sum2/1
  Sum2/1 -> Product5/2
  [A] -> Sum3/2
  Sum3/1 -> Product5/1
  Constant2/1 -> Sum3/1

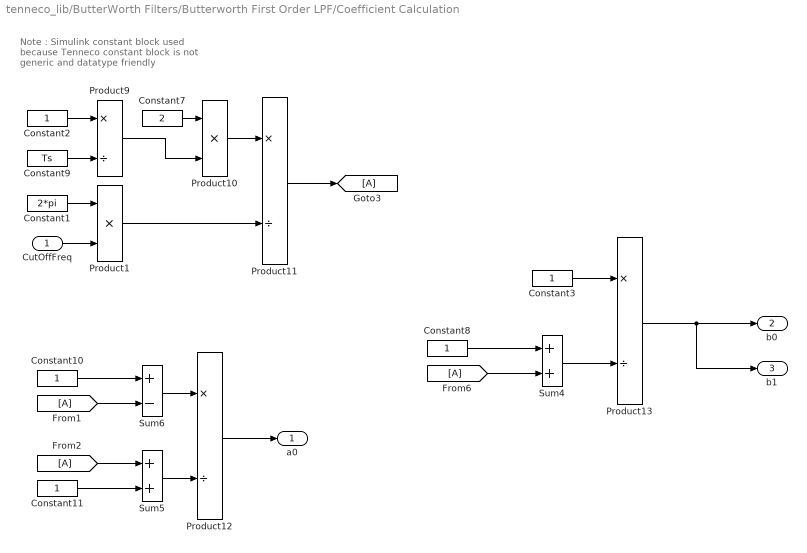
== system tenneco_lib/ButterWorth Filters/Butterworth First Order LPF/Coefficient Calculation ==
  note: Note : Simulink constant block used because Tenneco constant block is not generic and datatype friendly
  CutOffFreq : Inport  mask(Standard Inport){Port=1}
      mask prompts: Port "Simulink:blkprm_prompts:InOutportPortNum"
      mask help: Provide an input port for subsystems.
      mask TypeOptions Port: Port
  Constant1 : Constant  Value=2*pi  OutDataTypeStr=Inherit: Inherit via back propagation
  Constant{2..3,8,10..11} (5 alike) : Constant  OutDataTypeStr=Inherit: Inherit via back propagation
  Constant7 : Constant  Value=2  OutDataTypeStr=Inherit: Inherit via back propagation
  Constant9 : Constant  Value=Ts  OutDataTypeStr=Inherit: Inherit via back propagation
  Product1 : Product  Inputs=**  InputSameDT=on  mask(Product){Inputs=**}
      mask prompts: Inputs "List of signs:"
      mask help:
      | Multiply or divide inputs.  Specify one of the following:
      |  a) * or / for each input port. For example, **/* performs the operation 'u1*u2/u3*u4'.
      |  b) scalar specifies the number of input ports to be multiplied.
      mask TypeOptions Inputs: Inputs
  Product10 : Product  Inputs=**  InputSameDT=on  mask(Product){Inputs=**}
      mask prompts: Inputs "List of signs:"
      mask help:
      | Multiply or divide inputs.  Specify one of the following:
      |  a) * or / for each input port. For example, **/* performs the operation 'u1*u2/u3*u4'.
      |  b) scalar specifies the number of input ports to be multiplied.
      mask TypeOptions Inputs: Inputs
  Product11 : Product  Inputs=*/  InputSameDT=on  mask(Product){Inputs=*/}
      mask prompts: Inputs "List of signs:"
      mask help:
      | Multiply or divide inputs.  Specify one of the following:
      |  a) * or / for each input port. For example, **/* performs the operation 'u1*u2/u3*u4'.
      |  b) scalar specifies the number of input ports to be multiplied.
      mask TypeOptions Inputs: Inputs
  Product12 : Product  Inputs=*/  InputSameDT=on  mask(Product){Inputs=*/}
      mask prompts: Inputs "List of signs:"
      mask help:
      | Multiply or divide inputs.  Specify one of the following:
      |  a) * or / for each input port. For example, **/* performs the operation 'u1*u2/u3*u4'.
      |  b) scalar specifies the number of input ports to be multiplied.
      mask TypeOptions Inputs: Inputs
  Product13 : Product  Inputs=*/  InputSameDT=on  mask(Product){Inputs=*/}
      mask prompts: Inputs "List of signs:"
      mask help:
      | Multiply or divide inputs.  Specify one of the following:
      |  a) * or / for each input port. For example, **/* performs the operation 'u1*u2/u3*u4'.
      |  b) scalar specifies the number of input ports to be multiplied.
      mask TypeOptions Inputs: Inputs
  Product9 : Product  Inputs=*/  InputSameDT=on  mask(Product){Inputs=*/}
      mask prompts: Inputs "List of signs:"
      mask help:
      | Multiply or divide inputs.  Specify one of the following:
      |  a) * or / for each input port. For example, **/* performs the operation 'u1*u2/u3*u4'.
      |  b) scalar specifies the number of input ports to be multiplied.
      mask TypeOptions Inputs: Inputs
  Sum4 : Sum  InputSameDT=on  mask(Sum){Inputs=++}
      mask prompts: Inputs "Simulink:blkprm_prompts:SumListofSigns"
      mask help:
      | Add or subtract inputs.  Specify one of the following:
      | a) character vector containing + or - for each input port, | for spacer between ports (e.g. ++|-|++)
      | b) scalar, >= 1, specifies the number of input ports to be summed.
      | When there is only one input port, add or subtract elements over all dimensions or one specified dimension
      mask TypeOptions Inputs: Inputs
  Sum5 : Sum  InputSameDT=on  mask(Sum){Inputs=++}
      mask prompts: Inputs "Simulink:blkprm_prompts:SumListofSigns"
      mask help:
      | Add or subtract inputs.  Specify one of the following:
      | a) character vector containing + or - for each input port, | for spacer between ports (e.g. ++|-|++)
      | b) scalar, >= 1, specifies the number of input ports to be summed.
      | When there is only one input port, add or subtract elements over all dimensions or one specified dimension
      mask TypeOptions Inputs: Inputs
  Sum6 : Sum  Inputs=+-  InputSameDT=on  mask(Sum){Inputs=+-}
      mask prompts: Inputs "Simulink:blkprm_prompts:SumListofSigns"
      mask help:
      | Add or subtract inputs.  Specify one of the following:
      | a) character vector containing + or - for each input port, | for spacer between ports (e.g. ++|-|++)
      | b) scalar, >= 1, specifies the number of input ports to be summed.
      | When there is only one input port, add or subtract elements over all dimensions or one specified dimension
      mask TypeOptions Inputs: Inputs
  a0 : Outport  mask(Standard Outport){Port=1}
      mask prompts: Port "Simulink:blkprm_prompts:InOutportPortNum"
      mask help: Provide an output port for subsystems.
      mask TypeOptions Port: Port
  b0 : Outport  Port=2  mask(Standard Outport){Port=2}
      mask prompts: Port "Simulink:blkprm_prompts:InOutportPortNum"
      mask help: Provide an output port for subsystems.
      mask TypeOptions Port: Port
  b1 : Outport  Port=3  mask(Standard Outport){Port=3}
      mask prompts: Port "Simulink:blkprm_prompts:InOutportPortNum"
      mask help: Provide an output port for subsystems.
      mask TypeOptions Port: Port
  wires:
  Constant9/1 -> Product9/2
  CutOffFreq/1 -> Product1/2
  Constant2/1 -> Product9/1
  Constant1/1 -> Product1/1
  Product1/1 -> Product11/2
  Constant10/1 -> Sum6/1
  Sum6/1 -> Product12/1
  Product11/1 -> [A]
  [A] -> Sum6/2
  Sum5/1 -> Product12/2
  [A] -> Sum5/1
  Constant11/1 -> Sum5/2
  Product12/1 -> a0/1
  Constant3/1 -> Product13/1
  Sum4/1 -> Product13/2
  Constant8/1 -> Sum4/1
  [A] -> Sum4/2
  Product13/1 -> b1/1, b0/1
  Product10/1 -> Product11/1
  Product9/1 -> Product10/2
  Constant7/1 -> Product10/1
